simulink model "PI_controller"  (R2017a)
settings: Solver=VariableStepAuto  StartTime=0.0  StopTime=60  RelTol=1e-3
values from neighbouring files (symbols this model uses):
  Kc = 0.56    [PID_controller_params.m]    (also in PI_controller_params.m = 8)
  tau_1 = 3    [PI_controller_params.m]
  tau_2 = 0.5    [PI_controller_params.m]
settings Model: Creator=adityaaaap  LastModifiedBy=adityaaaap

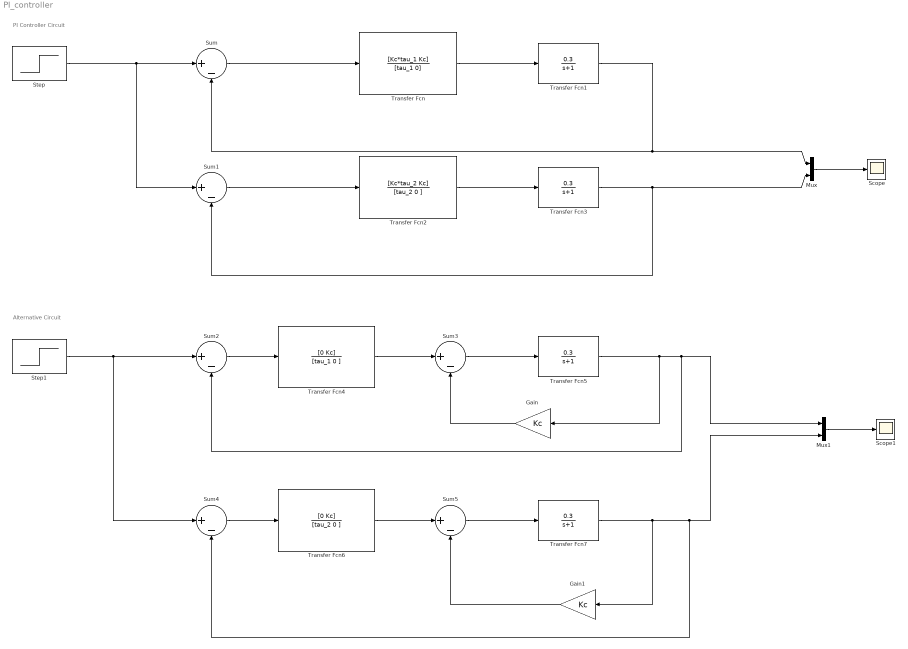
== system PI_controller ==
  note: Alternative Circuit
  note: PI Controller Circuit
  Gain : Gain  Gain=Kc
  Gain1 : Gain  Gain=Kc
  Mux : Mux  Inputs=2
  Mux1 : Mux  Inputs=2
  Scope : Scope
  Scope1 : Scope
  Step : Step  Time=0  SampleTime=0
  Step1 : Step  Time=0  SampleTime=0
  Sum{,1..5} (6 alike) : Sum  Inputs=|+-
  Transfer Fcn : TransferFcn  Numerator=[Kc*tau_1 Kc]  Denominator=[tau_1 0]
  Transfer Fcn{1,3,5,7} (4 alike) : TransferFcn  Numerator=[0.3]  Denominator=[1 1]
  Transfer Fcn2 : TransferFcn  Numerator=[Kc*tau_2 Kc]  Denominator=[tau_2 0 ]
  Transfer Fcn4 : TransferFcn  Numerator=[0 Kc]  Denominator=[tau_1 0 ]
  Transfer Fcn6 : TransferFcn  Numerator=[0 Kc]  Denominator=[tau_2 0 ]
  wires:
  Transfer Fcn/1 -> Transfer Fcn1/1
  Sum/1 -> Transfer Fcn/1
  Step/1 -> Sum1/1, Sum/1
  Transfer Fcn1/1 -> Sum/2, Mux/1
  Transfer Fcn2/1 -> Transfer Fcn3/1
  Sum1/1 -> Transfer Fcn2/1
  Transfer Fcn3/1 -> Mux/2, Sum1/2
  Mux/1 -> Scope/1
  Step1/1 -> Sum4/1, Sum2/1
  Sum2/1 -> Transfer Fcn4/1
  Transfer Fcn4/1 -> Sum3/1
  Sum3/1 -> Transfer Fcn5/1
  Transfer Fcn5/1 -> Gain/1, Sum2/2, Mux1/1
  Sum4/1 -> Transfer Fcn6/1
  Transfer Fcn6/1 -> Sum5/1
  Sum5/1 -> Transfer Fcn7/1
  Mux1/1 -> Scope1/1
  Transfer Fcn7/1 -> Gain1/1, Sum4/2, Mux1/2
  Gain/1 -> Sum3/2
  Gain1/1 -> Sum5/2
